simulink model "RT_ueb3_2c"  (R2013a)
settings: Solver=ode45  StartTime=0.0  StopTime=10.0  RelTol=1e-3
settings Model: BufferReuse=off  Creator=mainster  LastModifiedBy=mainster
settings OptimizationCC: InlineParams=on  BufferReuse=off
settings DebuggingCC: InitInArrayFormatMsg=none

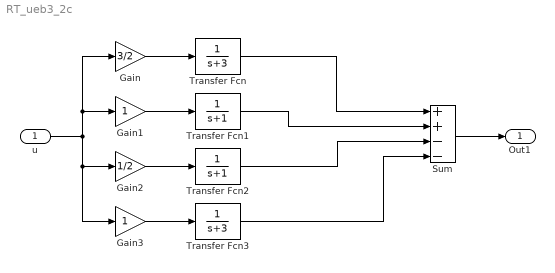
== system RT_ueb3_2c ==
  u : Inport
  Gain : Gain  Gain=3/2
  Gain1 : Gain
  Gain2 : Gain  Gain=1/2
  Gain3 : Gain
  Sum : Sum  Inputs=++--
  Transfer Fcn : TransferFcn  Denominator=[1 3]
  Transfer Fcn1 : TransferFcn  Denominator=[1 1]
  Transfer Fcn2 : TransferFcn  Denominator=[1 1]
  Transfer Fcn3 : TransferFcn  Denominator=[1 3]
  Out1 : Outport
  wires:
  Sum/1 -> Out1/1
  u/1 -> Gain3/1, Gain2/1, Gain1/1, Gain/1
  Gain/1 -> Transfer Fcn/1
  Transfer Fcn/1 -> Sum/1
  Gain1/1 -> Transfer Fcn1/1
  Transfer Fcn1/1 -> Sum/2
  Gain2/1 -> Transfer Fcn2/1
  Transfer Fcn2/1 -> Sum/3
  Gain3/1 -> Transfer Fcn3/1
  Transfer Fcn3/1 -> Sum/4
